simulink model "PIDbasic"  (Simulink 8.1)
settings: Solver=ode45  StartTime=0.0  StopTime=10.0  RelTol=1e-3
settings Model: Creator=eiseles  LastModifiedBy=eiseles
settings DataIOCC: SignalLoggingSaveFormat=Dataset
settings OptimizationCC: ExpressionDepthLimit=128
settings DebuggingCC: FcnCallInpInsideContextMsg=EnableAllAsError
settings GRTTargetCC: CombineOutputUpdateFcns=on  GRTInterface=off

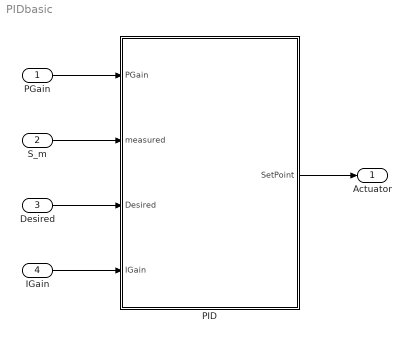
== system PIDbasic ==
  PGain : Inport
  S_m : Inport  Port=2
  Desired : Inport  Port=3
  IGain : Inport  Port=4
  PID : Subsystem
  Actuator : Outport
  wires:
  PID/1(SetPoint) -> Actuator/1
  Desired/1 -> PID/3(Desired)
  IGain/1 -> PID/4(IGain)
  PGain/1 -> PID/1(PGain)
  S_m/1 -> PID/2(measured)

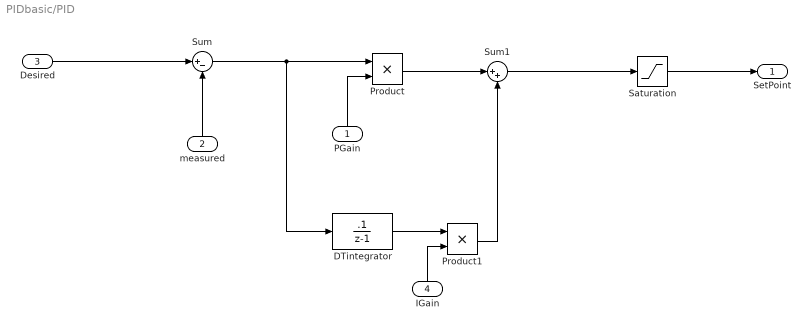
== system PIDbasic/PID ==
  PGain : Inport
  measured : Inport  Port=2
  Desired : Inport  Port=3
  IGain : Inport  Port=4
  DTintegrator : DiscreteTransferFcn  Numerator=[.1]  Denominator=[1 -1]  SampleTime=.1  a0EqualsOne=on
  Product : Product
  Product1 : Product
  Saturation : Saturate  UpperLimit=1  LowerLimit=-1
  Sum : Sum  Inputs=|+-
  Sum1 : Sum  Inputs=|++
  SetPoint : Outport
  wires:
  measured/1 -> Sum/2
  PGain/1 -> Product/2
  Saturation/1 -> SetPoint/1
  Product/1 -> Sum1/1
  DTintegrator/1 -> Product1/1
  IGain/1 -> Product1/2
  Product1/1 -> Sum1/2
  Sum/1 -> DTintegrator/1, Product/1
  Desired/1 -> Sum/1
  Sum1/1 -> Saturation/1
